simulink model "two_state_with_substates"  (R2017b)
settings: Solver=FixedStepDiscrete  StartTime=0.0  StopTime=10.0  RelTol=1e-3
settings Model: Creator=flosch  LastModifiedBy=flosch
settings ConfigComp: CovScope=ReferencedModels  CovIncludeTopModel=off

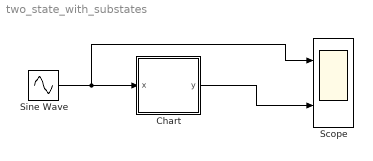
== system two_state_with_substates ==
  Chart : Stateflow chart  TreatAsAtomicUnit=on
  Scope : Scope  NumInputPorts=2
  Sine Wave : Sin  SampleTime=0
  wires:
  Sine Wave/1 -> Scope/1, Chart/1(x)
  Chart/1(y) -> Scope/2

== stateflow chart two_state_with_substates/Chart ==
  state Kitten
    entry: y = 0;
    state Foo
    state Bar
    (default) -> Foo
    Foo -> Bar : [x > 100]
    Bar -> Foo : [x < 90]
  state Potato
    entry: y = x;
  (default) -> Potato
  Kitten -> Potato : [x < t0]
  Potato -> Kitten : [x >= t0]
  data: t0 constant double =0.0; x input; y output
